simulink model "accrt"  (R2025a)
settings: Solver=FixedStepDiscrete  StartTime=0.0  StopTime=5.2  FixedStep=Ts  RelTol=1e-3
model workspace (MATLAB code in the model file):
  | N = 31;
  | n = 0:N-1;
  | sigma = (N-1)/6;
  | g = exp(-0.5*((n-(N-1)/2)/sigma).^2);
  | h = g / sum(g);
undefined symbols (not defined in the file): DiscIntNeverNeededParam, Ts
settings Model: Creator=wattanakhonvipanna  LastModifiedBy=wattanakhonvipanna

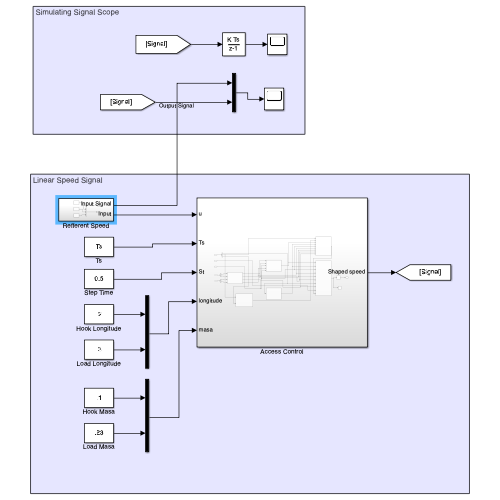
[thumbnail: Simulink's stored preview of the top-level diagram]
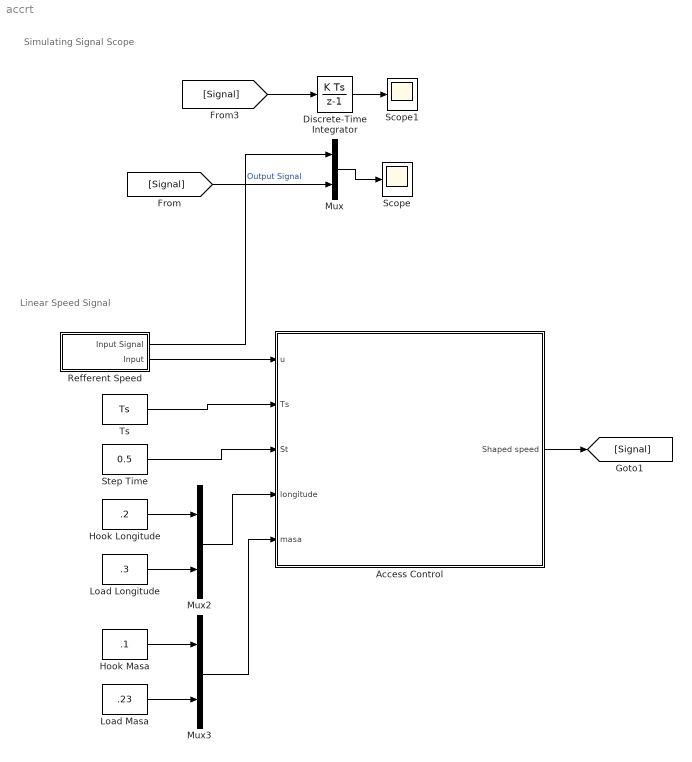
== system accrt ==
  note: Simulating Signal Scope
  note: Linear Speed Signal
  Access Control : Subsystem
  Discrete-Time Integrator : DiscreteIntegrator  SampleTime=-1  ICPrevOutput=DiscIntNeverNeededParam  ICPrevScaledInput=DiscIntNeverNeededParam
  Hook Longitude : Constant  Value=.2
  Hook Masa : Constant  Value=.1
  Load Longitude : Constant  Value=.3
  Load Masa : Constant  Value=.23
  Mux : Mux  Inputs=2
  Mux2 : Mux  Inputs=2
  Mux3 : Mux  Inputs=2
  Refferent Speed : Subsystem
  Scope : Scope
      settings: ActiveDisplayYMinimum=-0.024999999999999994  ActiveDisplayYMaximum=0.225  YLabel=speed (m/s)
  Scope1 : Scope
      settings: ActiveDisplayYMinimum=-0.0746290993622005  ActiveDisplayYMaximum=0.6716618942598046  YLabel=position (m)  DataLoggingVariableName=ScopeData2
  Step Time : Constant  Value=0.5
  Ts : Constant  Value=Ts
  wires:
  Step Time/1 -> Access Control/3(St)
  Mux/1 -> Scope/1
  Mux2/1 -> Access Control/4(longitude)
  Hook Longitude/1 -> Mux2/1
  Load Longitude/1 -> Mux2/2
  Load Masa/1 -> Mux3/2
  Hook Masa/1 -> Mux3/1
  Mux3/1 -> Access Control/5(masa)
  Discrete-Time Integrator/1 -> Scope1/1
  [Signal] -> Discrete-Time Integrator/1
  [Signal] -> Mux/2  "Output Signal"
  Access Control/1(Shaped speed) -> [Signal]
  Ts/1 -> Access Control/2(Ts)
  Refferent Speed/1(Input Signal) -> Mux/1
  Refferent Speed/2(Input) -> Access Control/1(u)

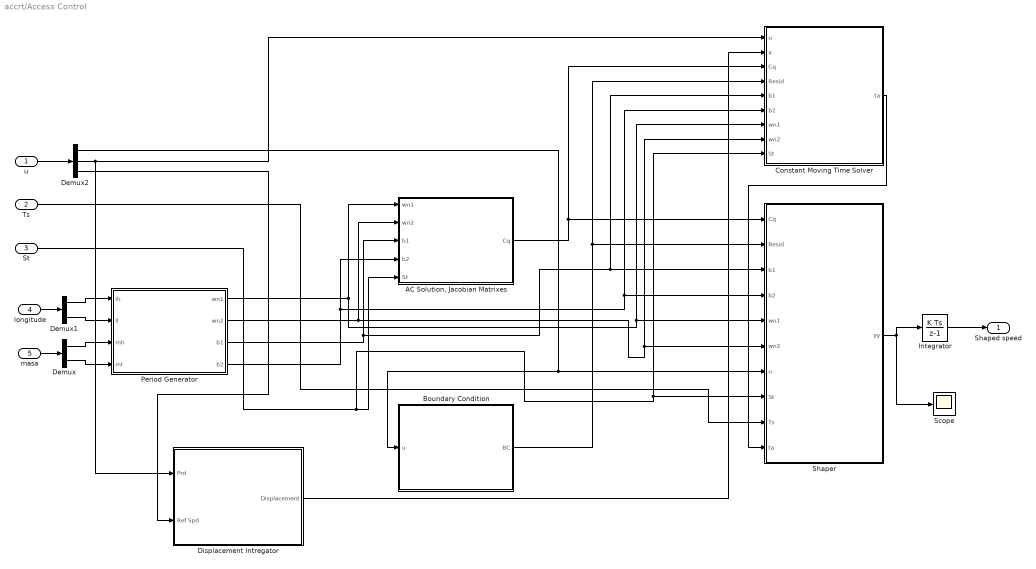
== system accrt/Access Control ==
  u : Inport
  Ts : Inport  Port=2
  St : Inport  Port=3
  longitude : Inport  Port=4
  masa : Inport  Port=5
  "AC Solution, Jacobian Matrixes" : MATLAB Function  TreatAsAtomicUnit=on
  Boundary Condition : MATLAB Function  TreatAsAtomicUnit=on
  Constant Moving Time Solver : MATLAB Function  TreatAsAtomicUnit=on
  Demux : Demux  Outputs=2
  Demux1 : Demux  Outputs=2
  Demux2 : Demux  Outputs=3
  Displacement Intregator : Subsystem
  Integrator : DiscreteIntegrator  SampleTime=-1  ICPrevOutput=DiscIntNeverNeededParam  ICPrevScaledInput=DiscIntNeverNeededParam
  Period Generator : MATLAB Function  TreatAsAtomicUnit=on
  Scope : Scope
      settings: ActiveDisplayYMinimum=-2.5086695159368269  ActiveDisplayYMaximum=2.5086695159368269
  Shaper : MATLAB Function  TreatAsAtomicUnit=on
  Shaped speed : Outport
  wires:
  masa/1 -> Demux/1
  longitude/1 -> Demux1/1
  Demux1/1 -> Period Generator/1(lh)
  Demux1/2 -> Period Generator/2(ll)
  Demux/1 -> Period Generator/3(mh)
  Demux/2 -> Period Generator/4(ml)
  "AC Solution, Jacobian Matrixes"/1(Cq) -> Constant Moving Time Solver/3(Cq), Shaper/1(Cq)
  Boundary Condition/1(BC) -> Constant Moving Time Solver/4(Resid), Shaper/2(Resid)
  Period Generator/4(b2) -> "AC Solution, Jacobian Matrixes"/4(b2), Constant Moving Time Solver/6(b2), Shaper/4(b2)
  Period Generator/3(b1) -> "AC Solution, Jacobian Matrixes"/3(b1), Constant Moving Time Solver/5(b1), Shaper/3(b1)
  Period Generator/2(wn2) -> Constant Moving Time Solver/8(wn2), Shaper/6(wn2), "AC Solution, Jacobian Matrixes"/2(wn2)
  Period Generator/1(wn1) -> "AC Solution, Jacobian Matrixes"/1(wn1), Constant Moving Time Solver/7(wn1), Shaper/5(wn1)
  St/1 -> "AC Solution, Jacobian Matrixes"/5(St), Constant Moving Time Solver/9(St), Shaper/8(St)
  Ts/1 -> Shaper/9(Ts)
  Shaper/1(yy) -> Integrator/1, Scope/1
  Integrator/1 -> Shaped speed/1
  Constant Moving Time Solver/1(ta) -> Shaper/10(ta)
  u/1 -> Demux2/1
  Demux2/1 -> Boundary Condition/1(u), Shaper/7(u)
  Demux2/3 -> Displacement Intregator/2(Ref Spd)
  Demux2/2 -> Constant Moving Time Solver/1(u), Displacement Intregator/1(Prd)
  Displacement Intregator/1(Displacement) -> Constant Moving Time Solver/2(x)

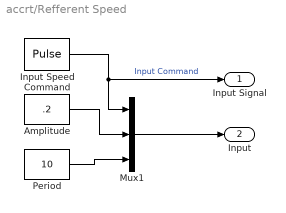
== system accrt/Refferent Speed ==
  Amplitude : Constant  Value=.2
  Input Speed Command : DiscretePulseGenerator  PulseType=Time based  Amplitude=.2  Period=10  PulseWidth=50
  Mux1 : Mux  Inputs=3
  Period : Constant  Value=10
  Input Signal : Outport
  Input : Outport  Port=2
  wires:
  Mux1/1 -> Input/1
  Amplitude/1 -> Mux1/2
  Period/1 -> Mux1/3
  Input Speed Command/1 -> Input Signal/1, Mux1/1  "Input Command"

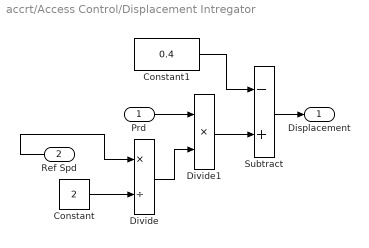
== system accrt/Access Control/Displacement Intregator ==
  Prd : Inport
  Ref Spd : Inport  Port=2
  Constant : Constant  Value=2
  Constant1 : Constant  Value=0.4
  Divide : Product  Inputs=*/
  Divide1 : Product  Inputs=**
  Subtract : Sum  Inputs=-+
  Displacement : Outport
  wires:
  Prd/1 -> Divide1/1
  Divide1/1 -> Subtract/2
  Subtract/1 -> Displacement/1
  Divide/1 -> Divide1/2
  Constant/1 -> Divide/2
  Ref Spd/1 -> Divide/1
  Constant1/1 -> Subtract/1

== matlab function accrt/Access Control/Period Generator ==
  data: lh input; ll input; mh input; wn1 output; wn2 output; ml input; b1 output; b2 output
function [wn1, wn2, b1, b2]= ModePeriodize(lh, ll, mh, ml)

g = 9.81;

M_s = [(mh+ml)*lh^2, ml*lh*ll; ml*lh*ll, ml*ll^2];
K_s = [(mh+ml)*g*lh, 0; 0, ml*g*ll];
B_s = [-(mh+ml)*lh; -ml*ll];

[mds_s,lambda_s] = eig(K_s,M_s);
omg_s = sqrt(diag(lambda_s));
b_nu_s = mds_s.'*B_s; 
wn1 = real(omg_s(1));
wn2 = real(omg_s(2));
b1 = real(b_nu_s(1));
b2 = real(b_nu_s(2));

== matlab function accrt/Access Control/Constant Moving Time Solver ==
  data: u input; x input; ta output; Cq input; Resid input; b1 input; b2 input; wn1 input; wn2 input; St input
function ta = findTa(u, x, Cq, Resid, b1, b2, wn1, wn2, St)

persistent armed  a1 a2 a3 a4 a5 a6 a7 a8 Tc d1 

if isempty(armed)
    armed  = false;

    a1=0; a2=0; a3=0; a4=0; a5=0; a6=0; a7=0; a8=0;
    Tc = 0;
    d1 = 0;
end

y   = 0;
ta = 0;


if ~armed 
    Tc    = St*2*pi/wn1;
    d1 = Tc;
    x = .6;
    C  = Cq \ Resid;
    a1 = C(1); a2 = C(2); a3 = C(3); a4 = C(4);
    a5 = C(5); a6 = C(6); a7 = C(7); a8 = C(8);

    armed = true;
end


if armed
   y = -1.0./wn1.^2.*(a1.*b1.*cos(wn1.*d1)+a2.*b1.*sin(wn1.*d1)) ...
       -1.0./wn2.^2.*(a3.*b2.*cos(wn2.*d1)+a4.*b2.*sin(wn2.*d1)) ...
       -(d1.^3.*(-a5+a2.*b1.*wn1+a4.*b2.*wn2))./6.0 ...
       -(d1.^2.*(-a6+a1.*b1+a3.*b2))./2.0 ...
       +1.0./wn1.^2.*1.0./wn2.^2.*(a8.*wn1.^2.*wn2.^2+a1.*b1.*wn2.^2+a3.*b2.*wn1.^2) ...
       +(d1.*(a2.*b1.*wn2+a4.*b2.*wn1+a7.*wn1.*wn2))./(wn1.*wn2);
   ta = (x - 2*y) / u;
   armed = false;
end
coder.extrinsic('assignin');
    assignin('base','A',[a1, a2, a3, a4, a5, a6, a7, a8]); 
    assignin('base','ta',ta); 
end

== matlab function accrt/Access Control/Boundary Condition ==
  data: u input; BC output
function BC = AcBC(u)
    velo_0 = 0.0;

    BC = [0.0; 0.0; 0.0; 0.0; 0.0;
             velo_0; 
             0.0; 0.0; 0.0; 0.0; 0.0; u];
end

== matlab function accrt/Access Control/AC Solution, Jacobian Matrixes ==
  data: wn1 input; wn2 input; Cq output; b1 input; b2 input; St input
function Cq = AcJacobian(wn1,wn2,b1,b2,St)
Tc = St*2*pi/wn1;
mt1 = [-b1.^2.*1.0./wn1.^2+(1.0./wn1.^3.*(b1.^2.*wn1.^3-b1.^2.*wn1.*wn2.^2))./((wn1+wn2).*(wn1-wn2)),-b1.*b2.*1.0./wn2.^2-(b1.*b2)./((wn1+wn2).*(wn1-wn2))+(b1.*b2.*wn1.^2.*1.0./wn2.^2)./((wn1+wn2).*(wn1-wn2)),0.0,0.0,0.0,0.0,-b1.^2.*1.0./wn1.^2+(1.0./wn1.^3.*(b1.^2.*wn1.^3.*cos(Tc.*wn1)-b1.^2.*wn1.*wn2.^2.*cos(Tc.*wn1)))./((wn1+wn2).*(wn1-wn2))+(Tc.*b1.^2.*sin(Tc.*wn1))./(wn1.*2.0)];
mt2 = [-b1.*b2.*1.0./wn2.^2-(b1.*b2.*cos(Tc.*wn1))./((wn1+wn2).*(wn1-wn2))+(b1.*b2.*wn1.^2.*1.0./wn2.^2.*cos(Tc.*wn2))./((wn1+wn2).*(wn1-wn2)),0.0,(b1.^2.*1.0./wn1.^2.*(wn1.*sin(Tc.*wn1)+Tc.*wn1.^2.*cos(Tc.*wn1)))./2.0-(1.0./wn1.^3.*(b1.^2.*wn1.^4.*sin(Tc.*wn1)-b1.^2.*wn1.^2.*wn2.^2.*sin(Tc.*wn1)))./((wn1+wn2).*(wn1-wn2)),(b1.*b2.*wn1.*sin(Tc.*wn1))./((wn1+wn2).*(wn1-wn2))-(b1.*b2.*wn1.^2.*sin(Tc.*wn2))./(wn2.*(wn1+wn2).*(wn1-wn2))];
mt3 = [-Tc.*b1+(b1.*sin(Tc.*wn1))./wn1,0.0,0.0,0.0,-b1.^2./wn1+(1.0./wn1.^3.*(b1.^2.*wn1.^4-b1.^2.*wn1.^2.*wn2.^2))./((wn1+wn2).*(wn1-wn2)),-b1.*b2.*wn1.*1.0./wn2.^2-(b1.*b2.*wn1)./((wn1+wn2).*(wn1-wn2))+(b1.*b2.*wn1.^3.*1.0./wn2.^2)./((wn1+wn2).*(wn1-wn2)),0.0];
mt4 = [-(Tc.*b1.^2)./wn1+(b1.^2.*1.0./wn1.^2.*(sin(Tc.*wn1)-Tc.*wn1.*cos(Tc.*wn1)))./2.0+(1.0./wn1.^3.*(b1.^2.*wn1.^3.*sin(Tc.*wn1)-b1.^2.*wn1.*wn2.^2.*sin(Tc.*wn1)))./((wn1+wn2).*(wn1-wn2)),-(b1.*b2.*sin(Tc.*wn1))./((wn1+wn2).*(wn1-wn2))-Tc.*b1.*b2.*wn1.*1.0./wn2.^2+(b1.*b2.*wn1.^3.*1.0./wn2.^3.*sin(Tc.*wn2))./((wn1+wn2).*(wn1-wn2)),b1.*wn1];
mt5 = [-b1.^2./wn1+(Tc.*b1.^2.*sin(Tc.*wn1))./2.0+(1.0./wn1.^3.*(b1.^2.*wn1.^4.*cos(Tc.*wn1)-b1.^2.*wn1.^2.*wn2.^2.*cos(Tc.*wn1)))./((wn1+wn2).*(wn1-wn2)),-b1.*b2.*wn1.*1.0./wn2.^2-(b1.*b2.*wn1.*cos(Tc.*wn1))./((wn1+wn2).*(wn1-wn2))+(b1.*b2.*wn1.^3.*1.0./wn2.^2.*cos(Tc.*wn2))./((wn1+wn2).*(wn1-wn2)),b1./wn1-(b1.*cos(Tc.*wn1))./wn1-(Tc.^2.*b1.*wn1)./2.0];
mt6 = [-b1.*b2.*1.0./wn1.^2+(b1.*b2)./((wn1+wn2).*(wn1-wn2))-(b1.*b2.*1.0./wn1.^2.*wn2.^2)./((wn1+wn2).*(wn1-wn2)),-b2.^2.*1.0./wn2.^2-(1.0./wn2.^3.*(b2.^2.*wn2.^3-b2.^2.*wn1.^2.*wn2))./((wn1+wn2).*(wn1-wn2)),0.0,0.0,0.0,0.0,-b1.*b2.*1.0./wn1.^2+(b1.*b2.*cos(Tc.*wn2))./((wn1+wn2).*(wn1-wn2))-(b1.*b2.*1.0./wn1.^2.*wn2.^2.*cos(Tc.*wn1))./((wn1+wn2).*(wn1-wn2))];
mt7 = [-b2.^2.*1.0./wn2.^2-(1.0./wn2.^3.*(b2.^2.*wn2.^3.*cos(Tc.*wn2)-b2.^2.*wn1.^2.*wn2.*cos(Tc.*wn2)))./((wn1+wn2).*(wn1-wn2))+(Tc.*b2.^2.*sin(Tc.*wn2))./(wn2.*2.0),0.0,-(b1.*b2.*wn2.*sin(Tc.*wn2))./((wn1+wn2).*(wn1-wn2))+(b1.*b2.*wn2.^2.*sin(Tc.*wn1))./(wn1.*(wn1+wn2).*(wn1-wn2))];
mt8 = [(b2.^2.*1.0./wn2.^2.*(wn2.*sin(Tc.*wn2)+Tc.*wn2.^2.*cos(Tc.*wn2)))./2.0+(1.0./wn2.^3.*(b2.^2.*wn2.^4.*sin(Tc.*wn2)-b2.^2.*wn1.^2.*wn2.^2.*sin(Tc.*wn2)))./((wn1+wn2).*(wn1-wn2)),-Tc.*b2+(b2.*sin(Tc.*wn2))./wn2,0.0,0.0,0.0,-b1.*b2.*1.0./wn1.^2.*wn2+(b1.*b2.*wn2)./((wn1+wn2).*(wn1-wn2))-(b1.*b2.*1.0./wn1.^2.*wn2.^3)./((wn1+wn2).*(wn1-wn2))];
mt9 = [-b2.^2./wn2-(1.0./wn2.^3.*(b2.^2.*wn2.^4-b2.^2.*wn1.^2.*wn2.^2))./((wn1+wn2).*(wn1-wn2)),0.0,(b1.*b2.*sin(Tc.*wn2))./((wn1+wn2).*(wn1-wn2))-Tc.*b1.*b2.*1.0./wn1.^2.*wn2-(b1.*b2.*1.0./wn1.^3.*wn2.^3.*sin(Tc.*wn1))./((wn1+wn2).*(wn1-wn2))];
mt10 = [-(Tc.*b2.^2)./wn2+(b2.^2.*1.0./wn2.^2.*(sin(Tc.*wn2)-Tc.*wn2.*cos(Tc.*wn2)))./2.0-(1.0./wn2.^3.*(b2.^2.*wn2.^3.*sin(Tc.*wn2)-b2.^2.*wn1.^2.*wn2.*sin(Tc.*wn2)))./((wn1+wn2).*(wn1-wn2)),b2.*wn2,-b1.*b2.*1.0./wn1.^2.*wn2+(b1.*b2.*wn2.*cos(Tc.*wn2))./((wn1+wn2).*(wn1-wn2))-(b1.*b2.*1.0./wn1.^2.*wn2.^3.*cos(Tc.*wn1))./((wn1+wn2).*(wn1-wn2))];
mt11 = [-b2.^2./wn2+(Tc.*b2.^2.*sin(Tc.*wn2))./2.0-(1.0./wn2.^3.*(b2.^2.*wn2.^4.*cos(Tc.*wn2)-b2.^2.*wn1.^2.*wn2.^2.*cos(Tc.*wn2)))./((wn1+wn2).*(wn1-wn2)),b2./wn2-(b2.*cos(Tc.*wn2))./wn2-(Tc.^2.*b2.*wn2)./2.0,0.0,0.0,0.0,b1.*1.0./wn1.^2-(1.0./wn1.^3.*(b1.*wn1.^3-b1.*wn1.*wn2.^2))./((wn1+wn2).*(wn1-wn2)),b2.*1.0./wn2.^2+(1.0./wn2.^3.*(b2.*wn2.^3-b2.*wn1.^2.*wn2))./((wn1+wn2).*(wn1-wn2)),0.0];
mt12 = [Tc.*b1.*1.0./wn1.^2-(1.0./wn1.^3.*(b1.*wn1.^2.*sin(Tc.*wn1)-b1.*wn2.^2.*sin(Tc.*wn1)))./((wn1+wn2).*(wn1-wn2)),Tc.*b2.*1.0./wn2.^2-(1.0./wn2.^3.*(b2.*wn1.^2.*sin(Tc.*wn2)-b2.*wn2.^2.*sin(Tc.*wn2)))./((wn1+wn2).*(wn1-wn2)),-1.0,b1.*1.0./wn1.^2-(1.0./wn1.^3.*(b1.*wn1.^3.*cos(Tc.*wn1)-b1.*wn1.*wn2.^2.*cos(Tc.*wn1)))./((wn1+wn2).*(wn1-wn2))];
mt13 = [b2.*1.0./wn2.^2+(1.0./wn2.^3.*(b2.*wn2.^3.*cos(Tc.*wn2)-b2.*wn1.^2.*wn2.*cos(Tc.*wn2)))./((wn1+wn2).*(wn1-wn2)),Tc.^2./2.0,b1.*1.0./wn1.^2-(1.0./wn1.^3.*(b1.*wn1.^3-b1.*wn1.*wn2.^2))./((wn1+wn2).*(wn1-wn2)),b2.*1.0./wn2.^2+(1.0./wn2.^3.*(b2.*wn2.^3-b2.*wn1.^2.*wn2))./((wn1+wn2).*(wn1-wn2)),0.0,0.0,0.0,0.0,b1.*1.0./wn1.^2-(1.0./wn1.^3.*(b1.*wn1.^3.*cos(Tc.*wn1)-b1.*wn1.*wn2.^2.*cos(Tc.*wn1)))./((wn1+wn2).*(wn1-wn2))];
mt14 = [b2.*1.0./wn2.^2+(1.0./wn2.^3.*(b2.*wn2.^3.*cos(Tc.*wn2)-b2.*wn1.^2.*wn2.*cos(Tc.*wn2)))./((wn1+wn2).*(wn1-wn2)),0.0,(1.0./wn1.^3.*(b1.*wn1.^4.*sin(Tc.*wn1)-b1.*wn1.^2.*wn2.^2.*sin(Tc.*wn1)))./((wn1+wn2).*(wn1-wn2)),-(1.0./wn2.^3.*(b2.*wn2.^4.*sin(Tc.*wn2)-b2.*wn1.^2.*wn2.^2.*sin(Tc.*wn2)))./((wn1+wn2).*(wn1-wn2)),Tc,0.0,0.0,0.0,0.0,0.0,1.0,0.0,0.0,0.0,0.0,0.0,1.0,0.0,0.0,1.0,0.0,0.0,0.0,0.0,0.0,0.0,0.0,0.0,0.0,0.0,0.0,0.0];
mt15 = [(1.0./wn1.^3.*(wn1.^5-wn1.^3.*wn2.^2))./((wn1+wn2).*(wn1-wn2)),0.0,0.0,(1.0./wn1.^3.*(wn1.^4.*sin(Tc.*wn1)-wn1.^2.*wn2.^2.*sin(Tc.*wn1)))./((wn1+wn2).*(wn1-wn2)),0.0,0.0,(1.0./wn1.^3.*(wn1.^5.*cos(Tc.*wn1)-wn1.^3.*wn2.^2.*cos(Tc.*wn1)))./((wn1+wn2).*(wn1-wn2)),0.0,0.0,(1.0./wn1.^3.*(wn1.^5-wn1.^3.*wn2.^2))./((wn1+wn2).*(wn1-wn2)),0.0,0.0,0.0,0.0,0.0];
mt16 = [(1.0./wn1.^3.*(wn1.^5.*cos(Tc.*wn1)-wn1.^3.*wn2.^2.*cos(Tc.*wn1)))./((wn1+wn2).*(wn1-wn2)),0.0,0.0,-(1.0./wn1.^3.*(wn1.^6.*sin(Tc.*wn1)-wn1.^4.*wn2.^2.*sin(Tc.*wn1)))./((wn1+wn2).*(wn1-wn2)),0.0,0.0,0.0,0.0,0.0,0.0,-(1.0./wn2.^3.*(wn2.^5-wn1.^2.*wn2.^3))./((wn1+wn2).*(wn1-wn2)),0.0,0.0,-(1.0./wn2.^3.*(wn2.^4.*sin(Tc.*wn2)-wn1.^2.*wn2.^2.*sin(Tc.*wn2)))./((wn1+wn2).*(wn1-wn2)),0.0,0.0];
mt17 = [-(1.0./wn2.^3.*(wn2.^5.*cos(Tc.*wn2)-wn1.^2.*wn2.^3.*cos(Tc.*wn2)))./((wn1+wn2).*(wn1-wn2)),0.0,0.0,-(1.0./wn2.^3.*(wn2.^5-wn1.^2.*wn2.^3))./((wn1+wn2).*(wn1-wn2)),0.0,0.0,0.0,0.0,0.0,-(1.0./wn2.^3.*(wn2.^5.*cos(Tc.*wn2)-wn1.^2.*wn2.^3.*cos(Tc.*wn2)))./((wn1+wn2).*(wn1-wn2)),0.0,0.0,(1.0./wn2.^3.*(wn2.^6.*sin(Tc.*wn2)-wn1.^2.*wn2.^4.*sin(Tc.*wn2)))./((wn1+wn2).*(wn1-wn2)),0.0];
Cq = reshape([mt1,mt2,mt3,mt4,mt5,mt6,mt7,mt8,mt9,mt10,mt11,mt12,mt13,mt14,mt15,mt16,mt17],12,12);

== matlab function accrt/Access Control/Shaper ==
  data: Cq input; yy output; Resid input; b1 input; b2 input; wn1 input; wn2 input; u input; St input; Ts input; ta input
function yy = ACshaped( Cq, Resid, b1, b2, wn1, wn2, u, St, Ts, ta)

persistent armed k a1 a2 a3 a4 a5 a6 last_u Tc d1 d2 yy_hist 

if isempty(armed)
    armed  = false;
    k      = 0;    
    a1=0; a2=0; a3=0; a4=0; a5=0; a6=0;
    last_u = 0; Tc = 0;
    d1 = 0; d2 = 0;
    yy_hist = zeros(1,1);
end

yy   = 0;
tol = 1e-12;

du     = u - last_u;
last_u = u;

if ~armed && (abs(du) > tol)
    Tc    = St*2*pi/wn1;
    k     = 0;
    d1 = round(Tc / Ts);
    d2 = round(ta / Ts); 

    C  = Cq \ Resid;
    a1 = C(1); a2 = C(2); a3 = C(3); a4 = C(4);
    a5 = C(5); a6 = C(6);

    yy_hist = zeros(1, d1);

    armed = true;
end

if armed
    t = double(k) * Ts;
    if k < d1
        yy = a6-t.*(-a5+a2.*b1.*wn1+a4.*b2.*wn2)-a1.*b1-a3.*b2+1.0./wn1.^2.* ...
            (a1.*b1.*wn1.^2.*cos(wn1.*t)+a2.*b1.*wn1.^2.*sin(wn1.*t))+1.0./wn2.^2.* ...
            (a3.*b2.*wn2.^2.*cos(wn2.*t)+a4.*b2.*wn2.^2.*sin(wn2.*t)) ; 
        yy_hist(k+1) = yy;
    elseif k > d1 && k <= d1+d2, yy = 0;
    elseif k > d1+d2 && k <= 2*d1+d2
        k_ref = k - (d1+d2);
        if k_ref <= length(yy_hist)
            yy = -yy_hist(k_ref);
        else
            yy = 0; 
        end
    end
    k = k + 1;
    if k > 2*d1+d2 +1
    armed = false;
    end
end
coder.extrinsic('assignin');
    assignin('base','a_vec',[Tc d2 Ts]);  
end
